simulink model "planRoadNetworkPath"  (R2024b)
settings: Solver=FixedStepAuto  StartTime=0.0  StopTime=10.0  RelTol=1e-3
settings Model: Creator=cstabile  LastModifiedBy=jbrault
settings SolverCC: DateTimeAtSimulationTimeZero=[]

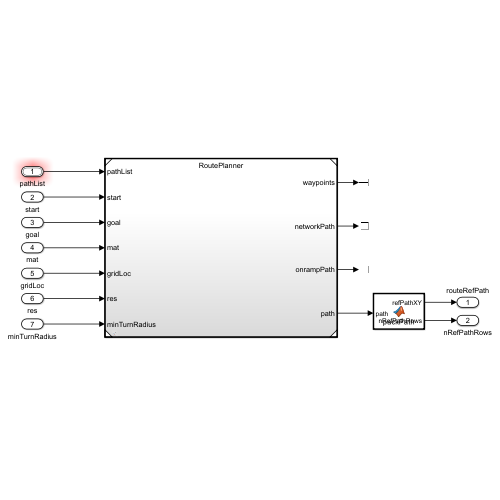
[thumbnail: Simulink's stored preview of the top-level diagram]
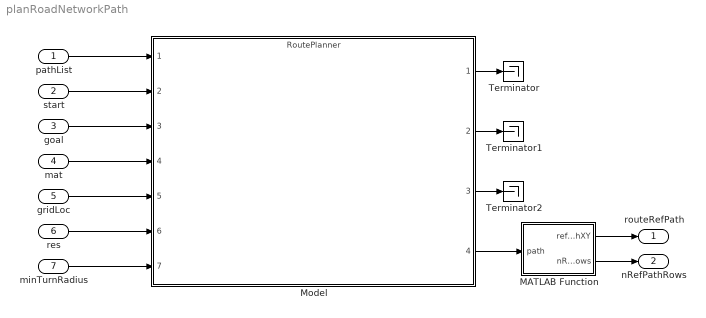
== system planRoadNetworkPath ==
  pathList : Inport  OutDataTypeStr=Bus: pathList_fixed_bus
  start : Inport  Port=2
  goal : Inport  Port=3
  mat : Inport  Port=4
  gridLoc : Inport  Port=5
  res : Inport  Port=6
  minTurnRadius : Inport  Port=7
  MATLAB Function : MATLAB Function  TreatAsAtomicUnit=on
  Model : ModelReference  ModelNameDialog=RoutePlanner.slx  SimulationMode=Normal  ModelReferenceVersion=3.0
  Terminator : Terminator
  Terminator1 : Terminator
  Terminator2 : Terminator
  routeRefPath : Outport
  nRefPathRows : Outport  Port=2
  wires:
  Model/1 -> Terminator/1
  MATLAB Function/1(refPathXY) -> routeRefPath/1
  minTurnRadius/1 -> Model/7
  Model/3 -> Terminator2/1
  MATLAB Function/2(nRefPathRows) -> nRefPathRows/1
  mat/1 -> Model/4
  Model/2 -> Terminator1/1
  start/1 -> Model/2
  pathList/1 -> Model/1
  Model/4 -> MATLAB Function/1(path)
  gridLoc/1 -> Model/5
  res/1 -> Model/6
  goal/1 -> Model/3

== matlab function planRoadNetworkPath/MATLAB Function ==
  data: path input; refPathXY output size=[1e4 3]; nRefPathRows output; maxRefPathLen parameter
function [refPathXY, nRefPathRows] = packPath(path, maxRefPathLen)

    % Allocate output buffer
    refPathXY = zeros(maxRefPathLen,3);
    nRefPathRows = size(path,1);
    refPathXY(1:nRefPathRows,:) = path;
end
